simulink model "mech_interface_dspring_damper"  (Simulink 7.1)
settings: Solver=ode15s  StartTime=0.0  StopTime=5  RelTol=1e-3
model workspace (MAT data in the model file):
  L_a = 1
  L_b = 1
  L_c = 0.1
  M_m = 0.5
  I_m : num (value not decoded)
PostLoadFcn:
  | hws = get_param(gcs, 'modelworkspace');
  | 
  | hws.assignin('L_a', 1);
  | hws.assignin('L_b', 1);
  | hws.assignin('L_c', 0.1);
  | 
  | hws.assignin('M_m', 0.5);
  | hws.evalin('I_m = [1/12*M_m*(L_b^2 + L_c^2) 0 0;   0 1/12*M_m*(L_a^2 + L_c^2) 0;   0 0 1/12*M_m*(L_a^2 + L_b^2)];');
  | 
  | clear hws
libraries: mblibv1 x17, fl_lib x6, nesl_utility x2
Description:
  | Mass Attached to Two Spring-Dampers
  | 
  | The model simulates a mass connected to ground by two spring-dampers. An initial force acts on the body for two seconds causing the body to oscillate. The Body Force Interface subsystems use Prismatic -Translational Interface blocks  with Spherical and Prismatic joints to connect each spring-damper between body and ground.
  | 
  | The spring-dampers and ground are modeled in Simscape. The rest of the mechanism is modeled in SimMechanics.
settings Model: Creator=ksanthan  LastModifiedBy=batserve
settings DataIOCC: OutputOption=SpecifiedOutputTimes  OutputTimes=[0:0.05:5]
settings DebuggingCC: AlgebraicLoopMsg=none  SaveWithParameterizedLinksMsg=none  SolverPrmCheckMsg=none
settings GRTTargetCC: TargetFcnLib=ansi_tfl_tmw.mat
settings SimMechanicsCC: VisOnUpdateDiagram=on  VisDuringSimulation=on

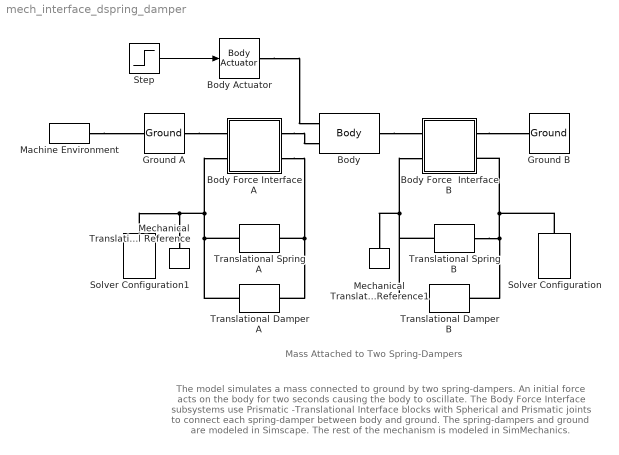
== system mech_interface_dspring_damper ==
  note: Mass Attached to Two Spring-Dampers
  note: The model simulates a mass connected to ground by two spring-dampers. An initial
      | force acts on the body for two seconds causing the body to oscillate. The Body Force Interface
      | subsystems use Prismatic -Translational Interface blocks  with Spherical and Prismatic joints
      | to connect each spring-damper between body and ground.
      |
      | The spring-dampers and ground are modeled in Simscape.
      | The rest of the mechanism is modeled in SimMechanics.
  Body : mblibv1/Bodies/Body  DialogController=MECH.DynMechDlgSource  PhysicalDomain=mechanical  SubClassName=Unknown  LeftPortType=workingframe  RightPortType=workingframe  LConnTagsString=CG|CS1  RConnTagsString=CS2  DialogClass=MechanicalBodyBlock  Mass=M_m  MassUnits=kg  InertiaUnits=kg*m^2  Inertia=I_m  Shape=Cylinder  ShapeDims=[1 1]  ShapeUnits=m  ShapeUse=false  Density=1  DensityUnits=kg/m^3  DensityUse=false  GraphicsMode=1  BodyColor=[0.5 0.5 0.5]  GraphicsObj=[]  AttachedToCS=1  CG=Left$CG$[L_a/2 0 0]$CS1$CS1$m$[0 0 0]$Euler X-Y-Z$deg$WORLD$true  WorkingFrames=Left$CS1$[0.0 0 0]$Adjoining$Adjoining$m$[0 0 0]$Euler X-Y-Z$deg$WORLD$true#Right$CS2$[L_a 0 0]$CS1$CS1$m$[0 0 0]$Euler X-Y-Z$deg$WORLD$true#Right$CS3$[L_a/2 -L_a/2 0]$CS1$CS1$m$[0 0 0]$Euler X-Y-Z$deg$WORLD$false#Right$CS4$[L_a/2 L_a/2 0]$CS1$CS1$m$[0 0 0]$Euler X-Y-Z$deg$WORLD$false  CGPos=[L_a/2 0 0]  CGRot=[0 0 0]  CS0Pos=[]  CS0Rot=[]  CS1Pos=[0.0 0 0]  CS1Rot=[0 0 0]  CS2Pos=[L_a 0 0]  CS2Rot=[0 0 0]  CS3Pos=[L_a/2 -L_a/2 0]  CS3Rot=[0 0 0]  CS4Pos=[L_a/2 L_a/2 0]  CS4Rot=[0 0 0]  CS5Pos=[]  CS5Rot=[]  CS6Pos=[]  CS6Rot=[]  CS7Pos=[]  CS7Rot=[]  CS8Pos=[]  CS8Rot=[]  CS9Pos=[]  CS9Rot=[]  CS10Pos=[]  CS10Rot=[]  CS11Pos=[]  CS11Rot=[]  CS12Pos=[]  CS12Rot=[]  CS13Pos=[]  CS13Rot=[]  CS14Pos=[]  CS14Rot=[]  CS15Pos=[]  CS15Rot=[]  CS16Pos=[]  CS16Rot=[]  CS17Pos=[]  CS17Rot=[]  CS18Pos=[]  CS18Rot=[]  CS19Pos=[]  CS19Rot=[]  CS20Pos=[]  CS20Rot=[]
  Body Actuator : mblibv1/Sensors &  Actuators/Body Actuator  DialogController=MECH.DynMechDlgSource  SystemSampleTime=-1  PhysicalDomain=Mechanical  PortType=blob  ActuationStyle=Force  AngleUnits=deg  ArcVelocityUnits=deg/s  ArcAccelerationUnits=deg/s^2  CoordPositionUnits=m  VelocityUnits=m/s  AccelerationUnits=m/s^2  ForceUnits=N  TorqueUnits=N*m  ActiveIO=on  Width=3  DialogClass=MechanicalActuatorBlock  ReferenceFrame=Absolute (World)  Angle=off  CoordPosition=on  Force=on  Torque=off
  Body Force  Interface B : Subsystem
  Body Force Interface A : Subsystem
  Ground A : mblibv1/Bodies/Ground  DialogController=MECH.DynMechDlgSource  SystemSampleTime=-1  LeftPortType=env  RightPortType=workingframe  PhysicalDomain=Mechanical  DialogClass=GroundBlock  CoordPosition=[0 0 0]  CoordPositionUnits=m  StateVectorMgrId=-1  MachineId=[0 0]  ShowEnvPort=on
  Ground B : mblibv1/Bodies/Ground  Orientation=left  DialogController=MECH.DynMechDlgSource  SystemSampleTime=-1  LeftPortType=env  RightPortType=workingframe  PhysicalDomain=Mechanical  DialogClass=GroundBlock  CoordPosition=[2 0 0]  CoordPositionUnits=m  StateVectorMgrId=-1  MachineId=[0 0]  ShowEnvPort=off
  Machine Environment : mblibv1/Bodies/Machine Environment  Tag=Factory ground  DialogController=MECH.DialogSource  SystemSampleTime=-1  PortType=env  PhysicalDomain=Mechanical  DialogTemplateClass=MECH.MachineEnvironment  SyncWhenCopied=off  Gravity=[0 0 0]  GravityUnits=m/s^2  GravityAsSignal=off  Dimensionality=Auto-detect  AnalysisType=Forward dynamics  LinearAssemblyTolerance=1e-3  LinearAssemblyToleranceUnits=m  AngularAssemblyTolerance=1e-3  AngularAssemblyToleranceUnits=rad  ConstraintSolverType=Stabilizing  ConstraintRelTolerance=1e-4  ConstraintAbsTolerance=1e-4  UseRobustSingularityHandling=off  RedundancyAnalysisToleranceType=Automatically select tolerance  RedundancyAnalysisTolerance=1e-14  StatePerturbationType=Fixed  PerturbationSize=1e-5  VisualizeMachine=on
  Mechanical Translational Reference : fl_lib/Mechanical/Translational Elements/Mechanical Translational Reference  Orientation=down  DialogController=NetworkEngine.DynNeDlgSource  SystemSampleTime=-1  LocalVarLogging=[]
  Mechanical Translational Reference1 : fl_lib/Mechanical/Translational Elements/Mechanical Translational Reference  Orientation=down  DialogController=NetworkEngine.DynNeDlgSource  SystemSampleTime=-1  LocalVarLogging=[]
  Solver Configuration : nesl_utility/Solver Configuration  Orientation=up  DialogController=NetworkEngine.DynNeUtilDlgSource  SystemSampleTime=-1  PhysicalDomain=network_engine_domain  LeftPortType=input  RightPortType=generic  SubClassName=solver  Accelerate=off  Profile=off  ResidualTolerance=1e-9  MaxNonlinIter=12  MaxModeIter=2  DoFixedCost=off  DoDC=off  LinearAlgebra=Sparse
  Solver Configuration1 : nesl_utility/Solver Configuration  Orientation=up  DialogController=NetworkEngine.DynNeUtilDlgSource  SystemSampleTime=-1  PhysicalDomain=network_engine_domain  LeftPortType=input  RightPortType=generic  SubClassName=solver  Accelerate=off  Profile=off  ResidualTolerance=1e-9  MaxNonlinIter=12  MaxModeIter=2  DoFixedCost=off  DoDC=off  LinearAlgebra=Sparse
  Step : Step  Time=2  Before=[50 50 0]  After=[0 0 0]  SampleTime=0
  Translational Damper A : fl_lib/Mechanical/Translational Elements/Translational Damper  Orientation=left  DialogController=NetworkEngine.DynNeDlgSource  SystemSampleTime=-1  D=100 N/(m/s)  force_Log=off  rel_velocity_Log=off  power_Log=off  LocalVarNames=|force|rel_velocity|power  LocalVarDescs=|Damping force (N)|Damper relative velocity (m/s)|Power dissipated in the damper (W)  LocalVarLogging=[0 0 0]
  Translational Damper B : fl_lib/Mechanical/Translational Elements/Translational Damper  Orientation=left  DialogController=NetworkEngine.DynNeDlgSource  SystemSampleTime=-1  D=100 N/(m/s)  force_Log=off  rel_velocity_Log=off  power_Log=off  LocalVarNames=|force|rel_velocity|power  LocalVarDescs=|Damping force (N)|Damper relative velocity (m/s)|Power dissipated in the damper (W)  LocalVarLogging=[0 0 0]
  Translational Spring A : fl_lib/Mechanical/Translational Elements/Translational Spring  Orientation=left  DialogController=NetworkEngine.DynNeDlgSource  SystemSampleTime=-1  spr_rate=100 N/m  init_def=0 m  force_Log=off  deformation_Log=off  LocalVarNames=|force|deformation  LocalVarDescs=|Spring force (N)|Spring deformation (m)  LocalVarLogging=[0 0]
  Translational Spring B : fl_lib/Mechanical/Translational Elements/Translational Spring  Orientation=left  DialogController=NetworkEngine.DynNeDlgSource  SystemSampleTime=-1  spr_rate=100 N/m  init_def=0 m  force_Log=off  deformation_Log=off  LocalVarNames=|force|deformation  LocalVarDescs=|Spring force (N)|Spring deformation (m)  LocalVarLogging=[0 0]
  wires:
  Step/1 -> Body Actuator/1
  connections:
  Machine Environment/RConn1 -- Ground A/LConn1
  Ground A/RConn1 -- Body Force Interface A/LConn1
  Body Force Interface A/RConn1 -- Body/LConn2
  Body/RConn1 -- Body Force  Interface B/LConn1
  Body Force  Interface B/RConn1 -- Ground B/RConn1
  Translational Spring A/RConn1 -- Body Force Interface A/LConn2 -- Mechanical Translational Reference/LConn1 -- Solver Configuration1/RConn1 -- Translational Damper A/RConn1
  Body Force Interface A/RConn2 -- Translational Spring A/LConn1 -- Translational Damper A/LConn1
  Translational Spring B/RConn1 -- Translational Damper B/RConn1 -- Body Force  Interface B/LConn2 -- Mechanical Translational Reference1/LConn1
  Translational Spring B/LConn1 -- Body Force  Interface B/RConn2 -- Solver Configuration/RConn1 -- Translational Damper B/LConn1
  Body Actuator/RConn1 -- Body/LConn1

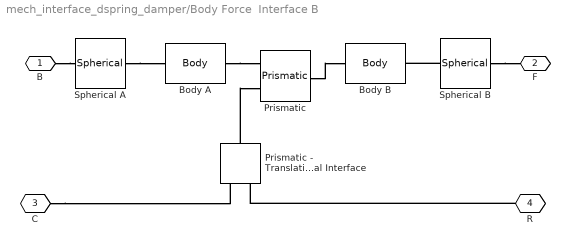
== system mech_interface_dspring_damper/Body Force  Interface B ==
  Body A : mblibv1/Bodies/Body  DialogController=MECH.DynMechDlgSource  PhysicalDomain=mechanical  SubClassName=Unknown  LeftPortType=workingframe  RightPortType=workingframe  LConnTagsString=CS1  RConnTagsString=CS2  DialogClass=MechanicalBodyBlock  Mass=1  MassUnits=kg  InertiaUnits=kg*m^2  Inertia=eye(3)*1e-4  Shape=Cylinder  ShapeDims=[1 1]  ShapeUnits=m  ShapeUse=false  Density=1  DensityUnits=kg/m^3  DensityUse=false  GraphicsMode=1  BodyColor=[0.5 0.5 0.5]  GraphicsObj=[]  AttachedToCS=1  CG=Left$CG$[-0.25 0 0]$CS2$CS2$m$[0 0 0]$Euler X-Y-Z$deg$WORLD$false  WorkingFrames=Left$CS1$[-0.5 0 0]$CS2$CS2$m$[0 0 0]$Euler X-Y-Z$deg$WORLD$true#Right$CS2$[0.5 0 0]$Adjoining$Adjoining$m$[0 0 0]$Euler X-Y-Z$deg$WORLD$true  CGPos=[-0.25 0 0]  CGRot=[0 0 0]  CS0Pos=[]  CS0Rot=[]  CS1Pos=[-0.5 0 0]  CS1Rot=[0 0 0]  CS2Pos=[0.5 0 0]  CS2Rot=[0 0 0]  CS3Pos=[]  CS3Rot=[]  CS4Pos=[]  CS4Rot=[]  CS5Pos=[]  CS5Rot=[]  CS6Pos=[]  CS6Rot=[]  CS7Pos=[]  CS7Rot=[]  CS8Pos=[]  CS8Rot=[]  CS9Pos=[]  CS9Rot=[]  CS10Pos=[]  CS10Rot=[]  CS11Pos=[]  CS11Rot=[]  CS12Pos=[]  CS12Rot=[]  CS13Pos=[]  CS13Rot=[]  CS14Pos=[]  CS14Rot=[]  CS15Pos=[]  CS15Rot=[]  CS16Pos=[]  CS16Rot=[]  CS17Pos=[]  CS17Rot=[]  CS18Pos=[]  CS18Rot=[]  CS19Pos=[]  CS19Rot=[]  CS20Pos=[]  CS20Rot=[]
  Body B : mblibv1/Bodies/Body  DialogController=MECH.DynMechDlgSource  PhysicalDomain=mechanical  SubClassName=Unknown  LeftPortType=workingframe  RightPortType=workingframe  LConnTagsString=CS1  RConnTagsString=CS2  DialogClass=MechanicalBodyBlock  Mass=1  MassUnits=kg  InertiaUnits=kg*m^2  Inertia=eye(3)*1e-4  Shape=Cylinder  ShapeDims=[1 1]  ShapeUnits=m  ShapeUse=false  Density=1  DensityUnits=kg/m^3  DensityUse=false  GraphicsMode=1  BodyColor=[0.5 0.5 0.5]  GraphicsObj=[]  AttachedToCS=1  CG=Left$CG$[-0.25 0 0]$CS2$CS2$m$[0 0 0]$Euler X-Y-Z$deg$WORLD$false  WorkingFrames=Left$CS1$[-0.5 0 0]$CS2$CS2$m$[0 0 0]$Euler X-Y-Z$deg$WORLD$true#Right$CS2$[0 0 0]$Adjoining$Adjoining$m$[0 0 0]$Euler X-Y-Z$deg$WORLD$true  CGPos=[-0.25 0 0]  CGRot=[0 0 0]  CS0Pos=[]  CS0Rot=[]  CS1Pos=[-0.5 0 0]  CS1Rot=[0 0 0]  CS2Pos=[0 0 0]  CS2Rot=[0 0 0]  CS3Pos=[]  CS3Rot=[]  CS4Pos=[]  CS4Rot=[]  CS5Pos=[]  CS5Rot=[]  CS6Pos=[]  CS6Rot=[]  CS7Pos=[]  CS7Rot=[]  CS8Pos=[]  CS8Rot=[]  CS9Pos=[]  CS9Rot=[]  CS10Pos=[]  CS10Rot=[]  CS11Pos=[]  CS11Rot=[]  CS12Pos=[]  CS12Rot=[]  CS13Pos=[]  CS13Rot=[]  CS14Pos=[]  CS14Rot=[]  CS15Pos=[]  CS15Rot=[]  CS16Pos=[]  CS16Rot=[]  CS17Pos=[]  CS17Rot=[]  CS18Pos=[]  CS18Rot=[]  CS19Pos=[]  CS19Rot=[]  CS20Pos=[]  CS20Rot=[]
  Prismatic : mblibv1/Joints/Prismatic  DialogController=MECH.DynMechDlgSource  PhysicalDomain=mechanical  SubClassName=Unknown  LeftPortType=blob  RightPortType=blob  LConnTagsString=__newl0|SA1  RConnTagsString=__newr0  NumSAPorts=1  CutJoint=off  MarkAsCut=off  Primitives=prismatic  PrimitiveProps=P1$Base$[1 0 0]$prismatic  DialogClass=JointBlock  P1Axis=[1 0 0]
  Prismatic - Translational Interface : mblibv1/Interface  Elements/Prismatic - Translational Interface  Orientation=up  DialogController=MECH.DynMechDlgSource  SystemSampleTime=-1  DialogClass=PrismaticTranslationalInterface  Primitive=P1
  "Spherical A " : mblibv1/Joints/Spherical  DialogController=MECH.DynMechDlgSource  PhysicalDomain=mechanical  SubClassName=Unknown  LeftPortType=blob  RightPortType=blob  LConnTagsString=__newl0  RConnTagsString=__newr0  NumSAPorts=0  CutJoint=off  MarkAsCut=off  Primitives=spherical  PrimitiveProps=S$WORLD$[0 0 0]$spherical  DialogClass=JointBlock  SAxis=[0 0 0]
  Spherical B : mblibv1/Joints/Spherical  DialogController=MECH.DynMechDlgSource  PhysicalDomain=mechanical  SubClassName=Unknown  LeftPortType=blob  RightPortType=blob  LConnTagsString=__newl0  RConnTagsString=__newr0  NumSAPorts=0  CutJoint=off  MarkAsCut=off  Primitives=spherical  PrimitiveProps=S$World$[0 0 0]$spherical  DialogClass=JointBlock  SAxis=[0 0 0]
  B : PMIOPort  Port=1  Side=Left
  F : PMIOPort  Orientation=left  Port=2  Side=Right
  C : PMIOPort  Port=3  Side=Left
  R : PMIOPort  Orientation=left  Port=4  Side=Right
  connections:
  Spherical B/RConn1 -- F/RConn1
  Spherical B/LConn1 -- Body B/RConn1
  R/RConn1 -- Prismatic - Translational Interface/LConn2
  C/RConn1 -- Prismatic - Translational Interface/LConn1
  B/RConn1 -- "Spherical A "/LConn1
  Prismatic/RConn1 -- Body B/LConn1
  Body A/RConn1 -- Prismatic/LConn1
  "Spherical A "/RConn1 -- Body A/LConn1
  Prismatic - Translational Interface/RConn1 -- Prismatic/LConn2

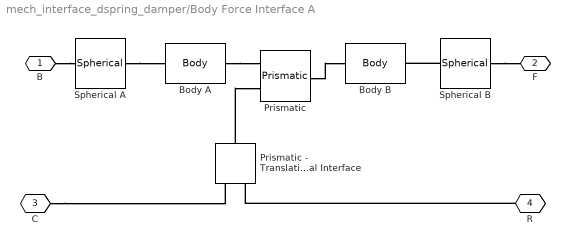
== system mech_interface_dspring_damper/Body Force Interface A ==
  Body A : mblibv1/Bodies/Body  DialogController=MECH.DynMechDlgSource  PhysicalDomain=mechanical  SubClassName=Unknown  LeftPortType=workingframe  RightPortType=workingframe  LConnTagsString=CS1  RConnTagsString=CS2  DialogClass=MechanicalBodyBlock  Mass=1  MassUnits=kg  InertiaUnits=kg*m^2  Inertia=eye(3)*1e-4  Shape=Cylinder  ShapeDims=[1 1]  ShapeUnits=m  ShapeUse=false  Density=1  DensityUnits=kg/m^3  DensityUse=false  GraphicsMode=1  BodyColor=[0.5 0.5 0.5]  GraphicsObj=[]  AttachedToCS=1  CG=Left$CG$[0.25 0 0]$CS1$CS1$m$[0 0 0]$Euler X-Y-Z$deg$WORLD$false  WorkingFrames=Left$CS1$[0 0 0]$Adjoining$Adjoining$m$[0 0 0]$Euler X-Y-Z$deg$WORLD$true#Right$CS2$[0.5 0 0]$CS1$CS1$m$[0 0 0]$Euler X-Y-Z$deg$WORLD$true  CGPos=[0.25 0 0]  CGRot=[0 0 0]  CS0Pos=[]  CS0Rot=[]  CS1Pos=[0 0 0]  CS1Rot=[0 0 0]  CS2Pos=[0.5 0 0]  CS2Rot=[0 0 0]  CS3Pos=[]  CS3Rot=[]  CS4Pos=[]  CS4Rot=[]  CS5Pos=[]  CS5Rot=[]  CS6Pos=[]  CS6Rot=[]  CS7Pos=[]  CS7Rot=[]  CS8Pos=[]  CS8Rot=[]  CS9Pos=[]  CS9Rot=[]  CS10Pos=[]  CS10Rot=[]  CS11Pos=[]  CS11Rot=[]  CS12Pos=[]  CS12Rot=[]  CS13Pos=[]  CS13Rot=[]  CS14Pos=[]  CS14Rot=[]  CS15Pos=[]  CS15Rot=[]  CS16Pos=[]  CS16Rot=[]  CS17Pos=[]  CS17Rot=[]  CS18Pos=[]  CS18Rot=[]  CS19Pos=[]  CS19Rot=[]  CS20Pos=[]  CS20Rot=[]
  Body B : mblibv1/Bodies/Body  DialogController=MECH.DynMechDlgSource  PhysicalDomain=mechanical  SubClassName=Unknown  LeftPortType=workingframe  RightPortType=workingframe  LConnTagsString=CS1  RConnTagsString=CS2  DialogClass=MechanicalBodyBlock  Mass=1  MassUnits=kg  InertiaUnits=kg*m^2  Inertia=eye(3)*1e-4  Shape=Cylinder  ShapeDims=[1 1]  ShapeUnits=m  ShapeUse=false  Density=1  DensityUnits=kg/m^3  DensityUse=false  GraphicsMode=1  BodyColor=[0.5 0.5 0.5]  GraphicsObj=[]  AttachedToCS=1  CG=Left$CG$[0.25 0 0]$CS1$CS1$m$[0 0 0]$Euler X-Y-Z$deg$WORLD$false  WorkingFrames=Left$CS1$[-0.5 0 0]$Adjoining$Adjoining$m$[0 0 0]$Euler X-Y-Z$deg$WORLD$true#Right$CS2$[0.5 0 0]$CS1$CS1$m$[0 0 0]$Euler X-Y-Z$deg$WORLD$true  CGPos=[0.25 0 0]  CGRot=[0 0 0]  CS0Pos=[]  CS0Rot=[]  CS1Pos=[-0.5 0 0]  CS1Rot=[0 0 0]  CS2Pos=[0.5 0 0]  CS2Rot=[0 0 0]  CS3Pos=[]  CS3Rot=[]  CS4Pos=[]  CS4Rot=[]  CS5Pos=[]  CS5Rot=[]  CS6Pos=[]  CS6Rot=[]  CS7Pos=[]  CS7Rot=[]  CS8Pos=[]  CS8Rot=[]  CS9Pos=[]  CS9Rot=[]  CS10Pos=[]  CS10Rot=[]  CS11Pos=[]  CS11Rot=[]  CS12Pos=[]  CS12Rot=[]  CS13Pos=[]  CS13Rot=[]  CS14Pos=[]  CS14Rot=[]  CS15Pos=[]  CS15Rot=[]  CS16Pos=[]  CS16Rot=[]  CS17Pos=[]  CS17Rot=[]  CS18Pos=[]  CS18Rot=[]  CS19Pos=[]  CS19Rot=[]  CS20Pos=[]  CS20Rot=[]
  Prismatic : mblibv1/Joints/Prismatic  DialogController=MECH.DynMechDlgSource  PhysicalDomain=mechanical  SubClassName=Unknown  LeftPortType=blob  RightPortType=blob  LConnTagsString=__newl0|SA1  RConnTagsString=__newr0  NumSAPorts=1  CutJoint=off  MarkAsCut=off  Primitives=prismatic  PrimitiveProps=P1$Base$[1 0 0]$prismatic  DialogClass=JointBlock  P1Axis=[1 0 0]
  Prismatic - Translational Interface : mblibv1/Interface  Elements/Prismatic - Translational Interface  Orientation=up  DialogController=MECH.DynMechDlgSource  SystemSampleTime=-1  DialogClass=PrismaticTranslationalInterface  Primitive=P1
  "Spherical A " : mblibv1/Joints/Spherical  DialogController=MECH.DynMechDlgSource  PhysicalDomain=mechanical  SubClassName=Unknown  LeftPortType=blob  RightPortType=blob  LConnTagsString=__newl0  RConnTagsString=__newr0  NumSAPorts=0  CutJoint=off  MarkAsCut=off  Primitives=spherical  PrimitiveProps=S$WORLD$[0 0 0]$spherical  DialogClass=JointBlock  SAxis=[0 0 0]
  Spherical B : mblibv1/Joints/Spherical  DialogController=MECH.DynMechDlgSource  PhysicalDomain=mechanical  SubClassName=Unknown  LeftPortType=blob  RightPortType=blob  LConnTagsString=__newl0  RConnTagsString=__newr0  NumSAPorts=0  CutJoint=off  MarkAsCut=off  Primitives=spherical  PrimitiveProps=S$World$[0 0 0]$spherical  DialogClass=JointBlock  SAxis=[0 0 0]
  B : PMIOPort  Port=1  Side=Left
  F : PMIOPort  Orientation=left  Port=2  Side=Right
  C : PMIOPort  Port=3  Side=Left
  R : PMIOPort  Orientation=left  Port=4  Side=Right
  connections:
  "Spherical A "/RConn1 -- Body A/LConn1
  Body A/RConn1 -- Prismatic/LConn1
  Prismatic/RConn1 -- Body B/LConn1
  Prismatic - Translational Interface/RConn1 -- Prismatic/LConn2
  B/RConn1 -- "Spherical A "/LConn1
  C/RConn1 -- Prismatic - Translational Interface/LConn1
  R/RConn1 -- Prismatic - Translational Interface/LConn2
  Spherical B/LConn1 -- Body B/RConn1
  Spherical B/RConn1 -- F/RConn1
